simulink model "multirotor_simulation"  (R2025b)
settings: Solver=ode4  StartTime=0.0  StopTime=21  FixedStep=ST  RelTol=1e-3
values from neighbouring files (symbols this model uses):
  a0 = 0    [multirotor_start.m]
  ASLOPE = 5.9    [multirotor_start.m]
  Ax = 0.023    [multirotor_start.m]
  Ay = 0.023    [multirotor_start.m]
  Az = 0.106    [multirotor_start.m]
  BLADES = 2    [multirotor_start.m]
  BLCG = 0    [multirotor_start.m]
  BLCP = 0    [multirotor_start.m]
  BLH1 = b*sind(30)    [multirotor_start.m]
  BLH2 = b    (= 0.275)    [multirotor_start.m]
  BLH3 = b*sind(30)    [multirotor_start.m]
  BLH4 = -b*sind(30)    [multirotor_start.m]
  BLH5 = -b    (= -0.275)    [multirotor_start.m]
  BLH6 = -b*sind(30)    [multirotor_start.m]
  chi1 = 1    [multirotor_start.m]
  chi2 = -1    [multirotor_start.m]
  chi3 = 1    [multirotor_start.m]
  chi4 = -1    [multirotor_start.m]
  chi5 = 1    [multirotor_start.m]
  chi6 = -1    [multirotor_start.m]
  CHORD = 17.55e-3    (= 0.01755)    [multirotor_start.m]
  CHORD75 = 21e-3    (= 0.021)    [multirotor_start.m]
  controller_mode = 1    [multirotor_start.m]
  del_sp = [0 0.7 0 0]'    [multirotor_start.m]
  dyn_visco = 17.89e-6    (= 1.789e-05)    [multirotor_start.m]
  g0 = 9.80665    [multirotor_start.m]
  href = 0    [multirotor_start.m]
  k_ind = 1.35    [multirotor_start.m]
  k_Omega = 14.92    [multirotor_start.m]
  latref = 44.200626    [multirotor_start.m]
  lonref = 12.063822    [multirotor_start.m]
  m = 2.15    [multirotor_start.m]
  MC_ATT_PITCH = 30*pi/180    (= 0.523598775598)    [multirotor_start.m]
  MC_ATT_ROLL = 30*pi/180    (= 0.523598775598)    [multirotor_start.m]
  MC_ATT_YAW = 180*pi/180    (= 3.14159265359)    [multirotor_start.m]
  MC_PITCH_P = 3    [multirotor_start.m]
  MC_PITCHRATE_D = 0    [multirotor_start.m]
  MC_PITCHRATE_I = 0.1*0.5    (= 0.05)    [multirotor_start.m]
  MC_PITCHRATE_P = 0.09    [multirotor_start.m]
  MC_ROLL_P = 3    [multirotor_start.m]
  MC_ROLLRATE_D = 0    [multirotor_start.m]
  MC_ROLLRATE_I = 0.1*0.5    (= 0.05)    [multirotor_start.m]
  MC_ROLLRATE_P = 0.09    [multirotor_start.m]
  MC_VEL_FWD = 5    [multirotor_start.m]
  MC_VEL_FWD_OPT = 0.5    [multirotor_start.m]
  MC_VEL_LAT = 5    [multirotor_start.m]
  MC_VEL_LAT_OPT = 0.5    [multirotor_start.m]
  MC_VEL_VERT = 1    [multirotor_start.m]
  MC_YAW_P = 1.8*0.5    (= 0.9)    [multirotor_start.m]
  MC_YAWRATE_D = 0    [multirotor_start.m]
  MC_YAWRATE_I = 0.1*0    (= 0)    [multirotor_start.m]
  MC_YAWRATE_P = 0.175*0.4    (= 0.07)    [multirotor_start.m]
  MPC_XY_VEL_D_ACC = 0.2*2    (= 0.4)    [multirotor_start.m]
  MPC_XY_VEL_I_ACC = 0.8    [multirotor_start.m]
  MPC_XY_VEL_P_ACC = 1.7*3/3    (= 1.7)    [multirotor_start.m]
  MPC_Z_VEL_D_ACC = 0    [multirotor_start.m]
  MPC_Z_VEL_I_ACC = 2    [multirotor_start.m]
  MPC_Z_VEL_P_ACC = 4    [multirotor_start.m]
  n = 0.6359    [multirotor_start.m]
  p00 = 7.145e-2    (= 0.07145)    [multirotor_start.m]
  p01 = 0.4377    [multirotor_start.m]
  p02 = -10.13    [multirotor_start.m]
  p10 = 1.259e-3    (= 0.001259)    [multirotor_start.m]
  p11 = 1.284e-3    (= 0.001284)    [multirotor_start.m]
  p20 = -7.513e-7    (= -7.513e-07)    [multirotor_start.m]
  PWM_hover = (PWM_idle+PWM_max)/2    (= 1550)    [multirotor_start.m]
  PWM_idle = 1100    [multirotor_start.m]
  PWM_max = 2000    [multirotor_start.m]
  ROTOR = 4*0.0254    (= 0.1016)    [multirotor_start.m]
  set_point_input = 0    [multirotor_start.m]
  ST = 0.01    [multirotor_start.m]
  STACG = 0    [multirotor_start.m]
  STACP = 0    [multirotor_start.m]
  STAH1 = -b*cosd(30)    [multirotor_start.m]
  STAH2 = 0    [multirotor_start.m]
  STAH3 = b*cosd(30)    [multirotor_start.m]
  STAH4 = b*cosd(30)    [multirotor_start.m]
  STAH5 = 0    [multirotor_start.m]
  STAH6 = -b*cosd(30)    [multirotor_start.m]
  TERMINAL_SPEED = 0.5    [multirotor_start.m]
  Theta0 = 45*pi/180    (= 0.785398163397)    [multirotor_start.m]
  THETT = -38.0973*pi/180    (= -0.66492332112)    [multirotor_start.m]
  V_sin_x = 0.3    [multirotor_start.m]
  Vsp = [0 1 0]'    [multirotor_start.m]
  wind_rate = [0 0 0]'    [multirotor_start.m]
  wind_velocity_e = [0 0 0]'    [multirotor_start.m]
  WLCG = -0.03    [multirotor_start.m]
  WLCP = -0.08    [multirotor_start.m]
  WLH1 = 32e-3    (= 0.032)    [multirotor_start.m]
  WLH2 = 32e-3    (= 0.032)    [multirotor_start.m]
  WLH3 = 32e-3    (= 0.032)    [multirotor_start.m]
  WLH4 = 32e-3    (= 0.032)    [multirotor_start.m]
  WLH5 = 32e-3    (= 0.032)    [multirotor_start.m]
  WLH6 = 32e-3    (= 0.032)    [multirotor_start.m]
  Xe_target = Xe_0 + [2, 3, -10]'    [multirotor_start.m]
undefined symbols (not defined in the file or in its folder): fspecial, gray, Rec, SDTV, Sim3dSensor, X, Y, Z
libraries: sm_lib x258, slpidlib x18, nesl_utility x15, sharedtransform x4, simulink x3, aerolibanimutils x2, sim3dcameralib x2, dspvision x2, uavsim3dlib x2, aerolibutil x2, visionconversions x1, visionanalysis x1
(part 10 of 10)

== matlab function multirotor_simulation/MULTIROTOR/MULTIPLE ROTORS FORCES AND MOMENTS/Subsystem3/MATLAB Function ==
  data: Q input; Pe output; Omega input; p00 input; p10 input; p01 input; p20 input; p11 input; p02 input
function Pe  = fcn(Q, Omega, p00, p10, p01, p20, p11, p02)
eta_e = p00 + p10*Omega  +p01*Q + p20*Omega^2 + p11*Omega*Q + p02*Q^2;
Psh = Omega*Q;
Pe=Psh/eta_e;

== matlab function multirotor_simulation/MULTIROTOR/MULTIPLE ROTORS FORCES AND MOMENTS/Subsystem3/NASA TM84281 ==
  data: BLADES input; F_rotor output; ASLOPE input; CHORD input; CHORD75 input; ROTOR input; a0 input; Theta0 input; THETT input; dyn_visco input; k_ind input; STACG input; BLCG input; WLCG input; STAH input; BLH input; WLH input; chi input; rho input; TAS input; omega_TAS input; Omega input; M_rotor output; Q output; vi output; lambda output; omega input; g input; h input
function [F_rotor, M_rotor, Q, vi, lambda] = fcn(BLADES, ASLOPE, CHORD, CHORD75, ROTOR, a0, Theta0, THETT, dyn_visco, k_ind, STACG, BLCG, WLCG, STAH, BLH, WLH, chi, rho, TAS, omega_TAS, Omega, omega, g, h)

%% Preliminary calculations
A = pi*ROTOR^2;
sigma = BLADES*CHORD/(pi*ROTOR);
lever_arm_H = [STACG-STAH BLH-BLCG WLCG-WLH]'; %STA-line and W-line against coordinate sys
TAS_H = [1 chi 1]'.*(TAS + cross(omega_TAS, lever_arm_H));
uH = TAS_H(1);
vH = TAS_H(2);
wH = TAS_H(3);
betta_w = atan2(vH, uH);
Mu = sqrt(uH^2+vH^2)/(Omega*ROTOR); %Ratio between the in -plane speed and the tip speed
p = omega(1); %Body Frame Roll-Rate
q = omega(2); %Body Frame Pitch-Ratw
pH = chi*p; %Hub Frame
qH = q; %Hub Frame
%Omega: scalar rate of rotor
%omega: rotation rate of MR

%% thrust calculations
lambda = fzero(@(x) x-wH/(Omega*ROTOR) + 0.5*((0.5*BLADES*rho*ASLOPE*CHORD*ROTOR*(Omega*ROTOR)^2*(x/2 + Theta0*(1/3+Mu^2/2) + THETT*(1/4+Mu^2/4) + Mu/4*(pH/Omega*cos(betta_w)+qH/Omega*sin(betta_w))))/(rho*A*(Omega*ROTOR)^2))/sqrt(Mu^2+x^2), -0.1);
T = (0.5*BLADES*rho*ASLOPE*CHORD*ROTOR*(Omega*ROTOR)^2*(lambda/2 + Theta0*(1/3+Mu^2/2) + THETT*(1/4+Mu^2/4) + Mu/4*(pH/Omega*cos(betta_w)+qH/Omega*sin(betta_w))));

%T = @(x)(0.5*BLADES*rho*ASLOPE*CHORD*ROTOR*(Omega*ROTOR)^2*(x/2 + Theta0*(1/3+Mu^2/2) + THETT*(1/4+Mu^2/4) + Mu/4*(pH/Omega*cos(betta_w)+qH/Omega*sin(betta_w))));
%lambda = fzero(@(x) x-wH/(Omega*ROTOR) + 0.5*(T(x)/(rho*A*(Omega*ROTOR)^2))/sqrt(Mu^2+x^2), -0.1);
%T = T(lambda);

vi = wH-lambda*Omega*ROTOR;

CT = T/(rho*A*(Omega*ROTOR)^2);
V75 = sqrt(vi^2+(0.75*Omega*ROTOR)^2);
Re = (rho*CHORD75*V75)/dyn_visco;
delta = 0.1166*Re^(-0.2) + 0.3/ASLOPE^2*(6*CT/sigma/(1+3/2*Mu^2))^2;

%% other forces and moments in the hub-wind frame
H_w=0.5*BLADES*rho*ASLOPE*CHORD*ROTOR*(Omega*ROTOR)^2 *((delta*Mu/(2*ASLOPE))-Theta0/4*(2*lambda*Mu +2/3*(pH/Omega *cos(betta_w) + qH/Omega *sin(betta_w))) - THETT/4*( Mu*lambda +0.5*(pH/Omega *cos(betta_w) + qH/Omega *sin(betta_w))) -0.25*(2/3*a0*(-pH/Omega *sin(betta_w)+ qH/Omega *cos(betta_w)) -2*lambda*(pH/Omega *cos(betta_w) + qH/Omega *sin(betta_w))) +0.25*Mu*a0^2);
Y_w=0.5*BLADES*rho*ASLOPE*CHORD*ROTOR*(Omega*ROTOR)^2 * (-0.25*Theta0*(3*a0*Mu- 2/3*(-pH/Omega *sin(betta_w)+qH/Omega *cos(betta_w))) -0.25*THETT*(2*a0*Mu -0.5*(-pH/Omega *sin(betta_w)+qH/Omega *cos(betta_w))) -0.25*6*Mu*a0*lambda);
L_w = 0;
M_w = 0;
Q=k_ind*(0.5*BLADES*rho*ASLOPE*CHORD*ROTOR^2*(Omega*ROTOR)^2*(delta/(4*ASLOPE*k_ind) *(1+Mu^2) -Theta0*(lambda/3 + Mu/6 *(pH/Omega *cos(betta_w) + qH/Omega *sin(betta_w))) -THETT*lambda*0.25 -0.5*(lambda^2 + Mu^2*(0.5*a0^2)) +Mu*a0/3*(-pH/Omega*sin(betta_w) +qH/Omega *cos(betta_w)) -1/8*(-pH/Omega*sin(betta_w) +qH/Omega *cos(betta_w))^2 -1/8*(pH/Omega *cos(betta_w) + qH/Omega *sin(betta_w))));

%% back rotation from hub-wind frame to hub frame
H_H = H_w*cos(betta_w) + Y_w*sin(betta_w);
Y_H = -H_w*sin(betta_w) + Y_w*cos(betta_w);
L_H = L_w*cos(betta_w) - M_w*sin(betta_w);
M_H = L_w*sin(betta_w) + M_w*cos(betta_w);

%% back rotation from hub frame to body frame
X = -H_H;
Y = chi*Y_H;
Z = -T;
F_rotor = [X Y Z]';
M_rotor = [chi*L_H M_H chi*Q]' + cross(lever_arm_H, F_rotor);

== matlab function multirotor_simulation/MULTIROTOR/MULTIPLE ROTORS FORCES AND MOMENTS/Subsystem4/MATLAB Function ==
  data: Q input; Pe output; Omega input; p00 input; p10 input; p01 input; p20 input; p11 input; p02 input
function Pe  = fcn(Q, Omega, p00, p10, p01, p20, p11, p02)
eta_e = p00 + p10*Omega  +p01*Q + p20*Omega^2 + p11*Omega*Q + p02*Q^2;
Psh = Omega*Q;
Pe=Psh/eta_e;

== matlab function multirotor_simulation/MULTIROTOR/MULTIPLE ROTORS FORCES AND MOMENTS/Subsystem4/NASA TM84281 ==
  data: BLADES input; F_rotor output; ASLOPE input; CHORD input; CHORD75 input; ROTOR input; a0 input; Theta0 input; THETT input; dyn_visco input; k_ind input; STACG input; BLCG input; WLCG input; STAH input; BLH input; WLH input; chi input; rho input; TAS input; omega_TAS input; Omega input; M_rotor output; Q output; vi output; lambda output; omega input; g input; h input
function [F_rotor, M_rotor, Q, vi, lambda] = fcn(BLADES, ASLOPE, CHORD, CHORD75, ROTOR, a0, Theta0, THETT, dyn_visco, k_ind, STACG, BLCG, WLCG, STAH, BLH, WLH, chi, rho, TAS, omega_TAS, Omega, omega, g, h)

%% Preliminary calculations
A = pi*ROTOR^2;
sigma = BLADES*CHORD/(pi*ROTOR);
lever_arm_H = [STACG-STAH BLH-BLCG WLCG-WLH]'; %STA-line and W-line against coordinate sys
TAS_H = [1 chi 1]'.*(TAS + cross(omega_TAS, lever_arm_H));
uH = TAS_H(1);
vH = TAS_H(2);
wH = TAS_H(3);
betta_w = atan2(vH, uH);
Mu = sqrt(uH^2+vH^2)/(Omega*ROTOR); %Ratio between the in -plane speed and the tip speed
p = omega(1); %Body Frame Roll-Rate
q = omega(2); %Body Frame Pitch-Ratw
pH = chi*p; %Hub Frame
qH = q; %Hub Frame
%Omega: scalar rate of rotor
%omega: rotation rate of MR

%% thrust calculations
lambda = fzero(@(x) x-wH/(Omega*ROTOR) + 0.5*((0.5*BLADES*rho*ASLOPE*CHORD*ROTOR*(Omega*ROTOR)^2*(x/2 + Theta0*(1/3+Mu^2/2) + THETT*(1/4+Mu^2/4) + Mu/4*(pH/Omega*cos(betta_w)+qH/Omega*sin(betta_w))))/(rho*A*(Omega*ROTOR)^2))/sqrt(Mu^2+x^2), -0.1);
T = (0.5*BLADES*rho*ASLOPE*CHORD*ROTOR*(Omega*ROTOR)^2*(lambda/2 + Theta0*(1/3+Mu^2/2) + THETT*(1/4+Mu^2/4) + Mu/4*(pH/Omega*cos(betta_w)+qH/Omega*sin(betta_w))));

%T = @(x)(0.5*BLADES*rho*ASLOPE*CHORD*ROTOR*(Omega*ROTOR)^2*(x/2 + Theta0*(1/3+Mu^2/2) + THETT*(1/4+Mu^2/4) + Mu/4*(pH/Omega*cos(betta_w)+qH/Omega*sin(betta_w))));
%lambda = fzero(@(x) x-wH/(Omega*ROTOR) + 0.5*(T(x)/(rho*A*(Omega*ROTOR)^2))/sqrt(Mu^2+x^2), -0.1);
%T = T(lambda);

vi = wH-lambda*Omega*ROTOR;

CT = T/(rho*A*(Omega*ROTOR)^2);
V75 = sqrt(vi^2+(0.75*Omega*ROTOR)^2);
Re = (rho*CHORD75*V75)/dyn_visco;
delta = 0.1166*Re^(-0.2) + 0.3/ASLOPE^2*(6*CT/sigma/(1+3/2*Mu^2))^2;

%% other forces and moments in the hub-wind frame
H_w=0.5*BLADES*rho*ASLOPE*CHORD*ROTOR*(Omega*ROTOR)^2 *((delta*Mu/(2*ASLOPE))-Theta0/4*(2*lambda*Mu +2/3*(pH/Omega *cos(betta_w) + qH/Omega *sin(betta_w))) - THETT/4*( Mu*lambda +0.5*(pH/Omega *cos(betta_w) + qH/Omega *sin(betta_w))) -0.25*(2/3*a0*(-pH/Omega *sin(betta_w)+ qH/Omega *cos(betta_w)) -2*lambda*(pH/Omega *cos(betta_w) + qH/Omega *sin(betta_w))) +0.25*Mu*a0^2);
Y_w=0.5*BLADES*rho*ASLOPE*CHORD*ROTOR*(Omega*ROTOR)^2 * (-0.25*Theta0*(3*a0*Mu- 2/3*(-pH/Omega *sin(betta_w)+qH/Omega *cos(betta_w))) -0.25*THETT*(2*a0*Mu -0.5*(-pH/Omega *sin(betta_w)+qH/Omega *cos(betta_w))) -0.25*6*Mu*a0*lambda);
L_w = 0;
M_w = 0;
Q=k_ind*(0.5*BLADES*rho*ASLOPE*CHORD*ROTOR^2*(Omega*ROTOR)^2*(delta/(4*ASLOPE*k_ind) *(1+Mu^2) -Theta0*(lambda/3 + Mu/6 *(pH/Omega *cos(betta_w) + qH/Omega *sin(betta_w))) -THETT*lambda*0.25 -0.5*(lambda^2 + Mu^2*(0.5*a0^2)) +Mu*a0/3*(-pH/Omega*sin(betta_w) +qH/Omega *cos(betta_w)) -1/8*(-pH/Omega*sin(betta_w) +qH/Omega *cos(betta_w))^2 -1/8*(pH/Omega *cos(betta_w) + qH/Omega *sin(betta_w))));

%% back rotation from hub-wind frame to hub frame
H_H = H_w*cos(betta_w) + Y_w*sin(betta_w);
Y_H = -H_w*sin(betta_w) + Y_w*cos(betta_w);
L_H = L_w*cos(betta_w) - M_w*sin(betta_w);
M_H = L_w*sin(betta_w) + M_w*cos(betta_w);

%% back rotation from hub frame to body frame
X = -H_H;
Y = chi*Y_H;
Z = -T;
F_rotor = [X Y Z]';
M_rotor = [chi*L_H M_H chi*Q]' + cross(lever_arm_H, F_rotor);

== matlab function multirotor_simulation/MULTIROTOR/MULTIPLE ROTORS FORCES AND MOMENTS/Subsystem5/MATLAB Function ==
  data: Q input; Pe output; Omega input; p00 input; p10 input; p01 input; p20 input; p11 input; p02 input
function Pe  = fcn(Q, Omega, p00, p10, p01, p20, p11, p02)
eta_e = p00 + p10*Omega  +p01*Q + p20*Omega^2 + p11*Omega*Q + p02*Q^2;
Psh = Omega*Q;
Pe=Psh/eta_e;

== matlab function multirotor_simulation/MULTIROTOR/MULTIPLE ROTORS FORCES AND MOMENTS/Subsystem5/NASA TM84281 ==
  data: BLADES input; F_rotor output; ASLOPE input; CHORD input; CHORD75 input; ROTOR input; a0 input; Theta0 input; THETT input; dyn_visco input; k_ind input; STACG input; BLCG input; WLCG input; STAH input; BLH input; WLH input; chi input; rho input; TAS input; omega_TAS input; Omega input; M_rotor output; Q output; vi output; lambda output; omega input; g input; h input
function [F_rotor, M_rotor, Q, vi, lambda] = fcn(BLADES, ASLOPE, CHORD, CHORD75, ROTOR, a0, Theta0, THETT, dyn_visco, k_ind, STACG, BLCG, WLCG, STAH, BLH, WLH, chi, rho, TAS, omega_TAS, Omega, omega, g, h)

%% Preliminary calculations
A = pi*ROTOR^2;
sigma = BLADES*CHORD/(pi*ROTOR);
lever_arm_H = [STACG-STAH BLH-BLCG WLCG-WLH]'; %STA-line and W-line against coordinate sys
TAS_H = [1 chi 1]'.*(TAS + cross(omega_TAS, lever_arm_H));
uH = TAS_H(1);
vH = TAS_H(2);
wH = TAS_H(3);
betta_w = atan2(vH, uH);
Mu = sqrt(uH^2+vH^2)/(Omega*ROTOR); %Ratio between the in -plane speed and the tip speed
p = omega(1); %Body Frame Roll-Rate
q = omega(2); %Body Frame Pitch-Ratw
pH = chi*p; %Hub Frame
qH = q; %Hub Frame
%Omega: scalar rate of rotor
%omega: rotation rate of MR

%% thrust calculations
lambda = fzero(@(x) x-wH/(Omega*ROTOR) + 0.5*((0.5*BLADES*rho*ASLOPE*CHORD*ROTOR*(Omega*ROTOR)^2*(x/2 + Theta0*(1/3+Mu^2/2) + THETT*(1/4+Mu^2/4) + Mu/4*(pH/Omega*cos(betta_w)+qH/Omega*sin(betta_w))))/(rho*A*(Omega*ROTOR)^2))/sqrt(Mu^2+x^2), -0.1);
T = (0.5*BLADES*rho*ASLOPE*CHORD*ROTOR*(Omega*ROTOR)^2*(lambda/2 + Theta0*(1/3+Mu^2/2) + THETT*(1/4+Mu^2/4) + Mu/4*(pH/Omega*cos(betta_w)+qH/Omega*sin(betta_w))));

%T = @(x)(0.5*BLADES*rho*ASLOPE*CHORD*ROTOR*(Omega*ROTOR)^2*(x/2 + Theta0*(1/3+Mu^2/2) + THETT*(1/4+Mu^2/4) + Mu/4*(pH/Omega*cos(betta_w)+qH/Omega*sin(betta_w))));
%lambda = fzero(@(x) x-wH/(Omega*ROTOR) + 0.5*(T(x)/(rho*A*(Omega*ROTOR)^2))/sqrt(Mu^2+x^2), -0.1);
%T = T(lambda);

vi = wH-lambda*Omega*ROTOR;

CT = T/(rho*A*(Omega*ROTOR)^2);
V75 = sqrt(vi^2+(0.75*Omega*ROTOR)^2);
Re = (rho*CHORD75*V75)/dyn_visco;
delta = 0.1166*Re^(-0.2) + 0.3/ASLOPE^2*(6*CT/sigma/(1+3/2*Mu^2))^2;

%% other forces and moments in the hub-wind frame
H_w=0.5*BLADES*rho*ASLOPE*CHORD*ROTOR*(Omega*ROTOR)^2 *((delta*Mu/(2*ASLOPE))-Theta0/4*(2*lambda*Mu +2/3*(pH/Omega *cos(betta_w) + qH/Omega *sin(betta_w))) - THETT/4*( Mu*lambda +0.5*(pH/Omega *cos(betta_w) + qH/Omega *sin(betta_w))) -0.25*(2/3*a0*(-pH/Omega *sin(betta_w)+ qH/Omega *cos(betta_w)) -2*lambda*(pH/Omega *cos(betta_w) + qH/Omega *sin(betta_w))) +0.25*Mu*a0^2);
Y_w=0.5*BLADES*rho*ASLOPE*CHORD*ROTOR*(Omega*ROTOR)^2 * (-0.25*Theta0*(3*a0*Mu- 2/3*(-pH/Omega *sin(betta_w)+qH/Omega *cos(betta_w))) -0.25*THETT*(2*a0*Mu -0.5*(-pH/Omega *sin(betta_w)+qH/Omega *cos(betta_w))) -0.25*6*Mu*a0*lambda);
L_w = 0;
M_w = 0;
Q=k_ind*(0.5*BLADES*rho*ASLOPE*CHORD*ROTOR^2*(Omega*ROTOR)^2*(delta/(4*ASLOPE*k_ind) *(1+Mu^2) -Theta0*(lambda/3 + Mu/6 *(pH/Omega *cos(betta_w) + qH/Omega *sin(betta_w))) -THETT*lambda*0.25 -0.5*(lambda^2 + Mu^2*(0.5*a0^2)) +Mu*a0/3*(-pH/Omega*sin(betta_w) +qH/Omega *cos(betta_w)) -1/8*(-pH/Omega*sin(betta_w) +qH/Omega *cos(betta_w))^2 -1/8*(pH/Omega *cos(betta_w) + qH/Omega *sin(betta_w))));

%% back rotation from hub-wind frame to hub frame
H_H = H_w*cos(betta_w) + Y_w*sin(betta_w);
Y_H = -H_w*sin(betta_w) + Y_w*cos(betta_w);
L_H = L_w*cos(betta_w) - M_w*sin(betta_w);
M_H = L_w*sin(betta_w) + M_w*cos(betta_w);

%% back rotation from hub frame to body frame
X = -H_H;
Y = chi*Y_H;
Z = -T;
F_rotor = [X Y Z]';
M_rotor = [chi*L_H M_H chi*Q]' + cross(lever_arm_H, F_rotor);

== matlab function multirotor_simulation/MULTIROTOR/MULTIPLE ROTORS FORCES AND MOMENTS/Subsystem/MATLAB Function ==
  data: Q input; Pe output; Omega input; p00 input; p10 input; p01 input; p20 input; p11 input; p02 input
function Pe  = fcn(Q, Omega, p00, p10, p01, p20, p11, p02)
eta_e = p00 + p10*Omega  +p01*Q + p20*Omega^2 + p11*Omega*Q + p02*Q^2;
Psh = Omega*Q;
Pe=Psh/eta_e;

== matlab function multirotor_simulation/MULTIROTOR/ESC + MOTOR/DJI OPTO 30A + DJI 2212 ==
  data: k_Omega input; Omega_array output; n input; PWM_idle input; PWM_array input
function Omega_array = fcn(k_Omega, n, PWM_idle, PWM_array)
delta = PWM_array-PWM_idle;       % if delta=0 => 0% Throttle
Omega_array = k_Omega*delta.^n;   % extrapolated function from experimental data points (only for spec. ESC+Motor)

== matlab function multirotor_simulation/PIXHAWK with PX4 Control System/ACCELLERATION AND YAW T ATTITUDE/MATLAB Function ==
  data: Asp input; theta_sp output; g0 input; psi_sp input; phi_sp output
function [theta_sp, phi_sp] = fcn(Asp, g0, psi_sp)
%first step: normalisatzion
I_e_cmd_z = (Asp-[0 0 g0]')/norm(Asp-[0 0 g0]');
%second step: first rotation to local frame
K_e_cmd_z = [cos(psi_sp) sin(psi_sp) 0; -sin(psi_sp) cos(psi_sp) 0; 0 0 1]*I_e_cmd_z;
%third step: extraction of remaining two angles (set point pitch and roll)
theta_sp = atan(K_e_cmd_z(1)/K_e_cmd_z(3));
phi_sp = atan(-1/cos(theta_sp)*K_e_cmd_z(2)*K_e_cmd_z(3)/(K_e_cmd_z(1)^2+K_e_cmd_z(3)^2));

== matlab function multirotor_simulation/PIXHAWK with PX4 Control System/ATTITUDE COONTROLLER/MATLAB Function ==
  data: qe input; Omegasp output; MC_ROLL_P input; MC_PITCH_P input; MC_YAW_P input
function Omegasp = fcn(qe, MC_ROLL_P, MC_PITCH_P, MC_YAW_P)
qe0 = qe(1);
qe1 = qe(2);
qe2 = qe(3);
qe3 = qe(4);

if qe0 >= 0
    s = 1;
else
    s = -1;
end
Omegasp = 2*s*[qe1*MC_ROLL_P; qe2*MC_PITCH_P; qe3*MC_YAW_P];

== matlab function multirotor_simulation/PIXHAWK with PX4 Control System/Motor Mixer ==
  data: PWM_vert input; PWM_array output; PWM_roll input; PWM_pitch input; PWM_yaw input
function PWM_array = fcn(PWM_vert, PWM_roll, PWM_pitch, PWM_yaw)
PWM_channels = [PWM_vert, PWM_roll, PWM_pitch, PWM_yaw]';
%MMmatrix = [1 -1 1 1; 1 -1 0 -1; 1 -1 -1 1; 1 1 -1 -1; 1 1 0 1; 1 1 1 -1];    %if rotor pushes more => effect on vert, roll, pitch, yaw
%MMmatrix = [1 -1 1 1; 1 -2 0 -1; 1 -1 -1 1; 1 1 -1 -1; 1 2 0 1; 1 1 1 -1];    %yaw correction, double contribution of rotor 2 and 5 on roll
MMmatrix = [1 -1 sqrt(3) 1; 1 -2 0 -1; 1 -1 -sqrt(3) 1; 1 1 -sqrt(3) -1; 1 2 0 1; 1 1 sqrt(3) -1];  %aggressiveness correction  3vs2 rotors
PWM_array = MMmatrix*PWM_channels;                                                                  %aggressivenis of roll and pich are same now
                                                                                                    %increase contrib. on pitch of all rotors except 0

== matlab function multirotor_simulation/PIXHAWK with PX4 Control System/VERTICAL CHANNEL CONTROLLER/MATLAB Function ==
  data: Asp input; delta_vert output; g0 input
function delta_vert = fcn(Asp, g0)
delta_vert = -Asp(3)/g0; %if going up, Asp(3) is negative

== matlab function multirotor_simulation/PIXHAWK with PX4 Control System/SPEED MAPPING FROM GCS/MATLAB Function1 ==
  data: pilot input; psisp input; Vsp_pilot output; MC_VEL_FWD input; MC_VEL_LAT input; MC_VEL_VERT input
function Vsp_pilot = fcn(pilot, psisp, MC_VEL_FWD, MC_VEL_LAT, MC_VEL_VERT)
Vsp_pilot_local = [-pilot(3)*MC_VEL_FWD, pilot(2)*MC_VEL_LAT, -pilot(1)*MC_VEL_VERT]'; %3rd input Pitch, 2nd input Roll, 1st input Throttle *conversion
%minus, to change joystick convention, on vert positive thrust = negative speed in ned frame
TLE = [cos(psisp) sin(psisp) 0; -sin(psisp) cos(psisp) 0; 0 0 1]; %rotation from local to inertial frame => joy in local => need Vsp in inertial
Vsp_pilot = TLE'*Vsp_pilot_local;

== matlab function multirotor_simulation/PIXHAWK with PX4 Control System/ATTITUDE MAPPING FROM GCS/MATLAB Function1 ==
  data: pilot input; eulersp_pilot output; MC_ATT_ROLL input; MC_ATT_PITCH input; MC_ATT_YAW input
function eulersp_pilot = fcn(pilot, MC_ATT_ROLL, MC_ATT_PITCH, MC_ATT_YAW)
eulersp_pilot = [pilot(2)*MC_ATT_ROLL pilot(3)*MC_ATT_PITCH pilot(4)*MC_ATT_YAW]';

== matlab function multirotor_simulation/Joy Stick // Interception/HUSKYLENS/VISION_DETECTION_SOFTWARE/Centroid Calculation ==
  data: Loc input; x_centroid output; y_centroid output; x_centroid_center output; y_centroid_center output
function [x_centroid, y_centroid, x_centroid_center, y_centroid_center] = fcn(Loc)
n = length(Loc(:,1));
x_centroid = round(1/n*sum(Loc(:,1))); %need integer
y_centroid = round(1/n*sum(Loc(:,2)));
x_centroid_center = round(x_centroid-640/2);
y_centroid_center = round(y_centroid-640/2);

== matlab function multirotor_simulation/PIXHAWK with PX4 Control System/OPTICAL_GUIDANCE_SYS (PROPORTIONAL)/MATLAB Function1 ==
  data: centroid_center input; psi input; Vsp_optical output; MC_VEL_FWD input; MC_VEL_LAT input; TERMINAL_SPEED input
function Vsp_optical = fcn(centroid_center, psi, MC_VEL_FWD, MC_VEL_LAT, TERMINAL_SPEED)
TLE = [cos(psi) sin(psi) 0; -sin(psi) cos(psi) 0; 0 0 1]; %From local in inertial
delta_roll = centroid_center(1)/320;    %normalization => [-1,1]
delta_pitch = centroid_center(2)/320;
Vsp_optical_local = [MC_VEL_FWD*delta_pitch MC_VEL_LAT*delta_roll -TERMINAL_SPEED]'; %minus bc ned => up
Vsp_optical = TLE'*Vsp_optical_local;

== matlab function multirotor_simulation/PIXHAWK with PX4 Control System/SPEED SP FROM SCRIPT/MATLAB Function ==
  data: v_sp input; v_sp_out output; sin_x input; V_sin_x input
function v_sp_out = fcn(v_sp, sin_x, V_sin_x)

v_sp_out = v_sp;
if V_sin_x ~= 0
    v_sp_out(1) = sin_x;
end

== matlab function multirotor_simulation/MULTIROTOR/FRAME/MATLAB Function ==
  data: Ax input; F_frame output; Ay input; Az input; STACP input; BLCP input; WLCP input; STACG input; BLCG input; WLCG input; rho input; TAS input; M_frame output
function [F_frame, M_frame] = fcn(Ax, Ay, Az, STACP, BLCP, WLCP, STACG, BLCG, WLCG, rho, TAS)
lever_arm_cp = [STACG-STACP BLCP-BLCG WLCG-WLCP]';
F_frame = -0.5*rho*[TAS(1)*Ax TAS(2)*Ay TAS(3)*Az]'*norm(TAS);
M_frame = cross(lever_arm_cp, F_frame);

== matlab function multirotor_simulation/MULTIROTOR/MULTIPLE ROTORS FORCES AND MOMENTS/Subsystem/NASA TM84281 ==
  data: BLADES input; F_rotor output; ASLOPE input; CHORD input; CHORD75 input; ROTOR input; a0 input; Theta0 input; THETT input; dyn_visco input; k_ind input; STACG input; BLCG input; WLCG input; STAH input; BLH input; WLH input; chi input; rho input; TAS input; omega_TAS input; Omega input; M_rotor output; Q output; vi output; lambda output; omega input; g input; h input
function [F_rotor, M_rotor, Q, vi, lambda] = fcn(BLADES, ASLOPE, CHORD, CHORD75, ROTOR, a0, Theta0, THETT, dyn_visco, k_ind, STACG, BLCG, WLCG, STAH, BLH, WLH, chi, rho, TAS, omega_TAS, Omega, omega, g, h)

%% Preliminary calculations
A = pi*ROTOR^2;
sigma = BLADES*CHORD/(pi*ROTOR);
lever_arm_H = [STACG-STAH BLH-BLCG WLCG-WLH]'; %STA-line and W-line against coordinate sys
TAS_H = [1 chi 1]'.*(TAS + cross(omega_TAS, lever_arm_H)); %TAS of Hub => translation + rotation
uH = TAS_H(1); %TAS components
vH = TAS_H(2);
wH = TAS_H(3);
betta_w = atan2(vH, uH); %Rotation from Hub to Wind frame
Mu = sqrt(uH^2+vH^2)/(Omega*ROTOR); %Ratio between the in -plane speed and the tip speed (advance ratio)
p = omega(1); %Body Frame Roll-Rate
q = omega(2); %Body Frame Pitch-Ratw
pH = chi*p; %Hub Frame => Assumption: tilt angle=0
qH = q; %Hub Frame
%Omega: scalar rate of rotor
%omega: rotation rate of MR

%% thrust calculations
lambda = fzero(@(x) x-wH/(Omega*ROTOR) + 0.5*((0.5*BLADES*rho*ASLOPE*CHORD*ROTOR*(Omega*ROTOR)^2*(x/2 + Theta0*(1/3+Mu^2/2) + THETT*(1/4+Mu^2/4) + Mu/4*(pH/Omega*cos(betta_w)+qH/Omega*sin(betta_w))))/(rho*A*(Omega*ROTOR)^2))/sqrt(Mu^2+x^2), -0.1);
T = (0.5*BLADES*rho*ASLOPE*CHORD*ROTOR*(Omega*ROTOR)^2*(lambda/2 + Theta0*(1/3+Mu^2/2) + THETT*(1/4+Mu^2/4) + Mu/4*(pH/Omega*cos(betta_w)+qH/Omega*sin(betta_w))));

vi = wH-lambda*Omega*ROTOR;

CT = T/(rho*A*(Omega*ROTOR)^2);
V75 = sqrt(vi^2+(0.75*Omega*ROTOR)^2);
Re = (rho*CHORD75*V75)/dyn_visco;
delta = 0.1166*Re^(-0.2) + 0.3/ASLOPE^2*(6*CT/sigma/(1+3/2*Mu^2))^2;   %Drag coefficient = \bar{c_d}

%% other forces and moments in the hub-wind frame %epsilon=0 eccentricity of blades
%we have very simple equations, bc EPSI=0 => excentricity
H_w=0.5*BLADES*rho*ASLOPE*CHORD*ROTOR*(Omega*ROTOR)^2 *((delta*Mu/(2*ASLOPE))-Theta0/4*(2*lambda*Mu +2/3*(pH/Omega *cos(betta_w) + qH/Omega *sin(betta_w))) - THETT/4*( Mu*lambda +0.5*(pH/Omega *cos(betta_w) + qH/Omega *sin(betta_w))) -0.25*(2/3*a0*(-pH/Omega *sin(betta_w)+ qH/Omega *cos(betta_w)) -2*lambda*(pH/Omega *cos(betta_w) + qH/Omega *sin(betta_w))) +0.25*Mu*a0^2);
Y_w=0.5*BLADES*rho*ASLOPE*CHORD*ROTOR*(Omega*ROTOR)^2 * (-0.25*Theta0*(3*a0*Mu- 2/3*(-pH/Omega *sin(betta_w)+qH/Omega *cos(betta_w))) -0.25*THETT*(2*a0*Mu -0.5*(-pH/Omega *sin(betta_w)+qH/Omega *cos(betta_w))) -0.25*6*Mu*a0*lambda);

L_w = 0;
M_w = 0;
Q=k_ind*(0.5*BLADES*rho*ASLOPE*CHORD*ROTOR^2*(Omega*ROTOR)^2*(delta/(4*ASLOPE*k_ind) *(1+Mu^2) -Theta0*(lambda/3 + Mu/6 *(pH/Omega *cos(betta_w) + qH/Omega *sin(betta_w))) -THETT*lambda*0.25 -0.5*(lambda^2 + Mu^2*(0.5*a0^2)) +Mu*a0/3*(-pH/Omega*sin(betta_w) +qH/Omega *cos(betta_w)) -1/8*(-pH/Omega*sin(betta_w) +qH/Omega *cos(betta_w))^2 -1/8*(pH/Omega *cos(betta_w) + qH/Omega *sin(betta_w))));
% Q = k_ind*(Q_id + Q_pr/k_ind)

%% back rotation from hub-wind frame to hub frame
H_H = H_w*cos(betta_w) + Y_w*sin(betta_w);
Y_H = -H_w*sin(betta_w) + Y_w*cos(betta_w);

L_H = L_w*cos(betta_w) - M_w*sin(betta_w);
M_H = L_w*sin(betta_w) + M_w*cos(betta_w);

%% back rotation from hub frame to body frame
X = -H_H;
Y = chi*Y_H;
Z = -T;
F_rotor = [X Y Z]';
M_rotor = [chi*L_H M_H chi*Q]' + cross(lever_arm_H, F_rotor); %correction term => change the reduction Pole,, Transportation of Moments
